simulink library "Solar_Radiation_Sensor"  (R2018b)
settings: Solver=ode45  StartTime=0.0  StopTime=10.0  RelTol=1e-3  EnableMultiTasking=on
settings Model: Creator=lena.frank  LastModifiedBy=P41573
settings DataIOCC: LimitDataPoints=on  SaveFormat=Array  SignalLoggingSaveFormat=ModelDataLogs
settings OptimizationCC: ExpressionDepthLimit=2147483647  LifeSpan=inf
settings DebuggingCC: UnderspecifiedInitializationDetection=Classic  MergeDetectMultiDrivingBlocksExec=none  SolverPrmCheckMsg=warning  FcnCallInpInsideContextMsg=warning  StateNameClashWarn=warning  SFUnexpectedBacktrackingDiag=warning  SFNoUnconditionalDefaultTransitionDiag=warning  SFExecutionAtInitializationDiag=none
settings HardwareCC: ProdBitPerPointer=32  ProdBitPerSizeT=32  ProdBitPerPtrDiffT=32  ProdLargestAtomicFloat=None  ProdIntDivRoundTo=Undefined  ProdEndianess=Unspecified  ProdWordSize=32  ProdHWDeviceType=32-bit Generic
settings ModelReferenceCC: PropagateSignalLabelsOutOfModel=off
settings SFSimCC: SimUseLocalCustomCode=off
settings RTWCC: RTWUseLocalCustomCode=off
settings CodeAppCC: StateflowObjectComments=on
settings GRTTargetCC: TargetLangStandard=C89/C90 (ANSI)  GeneratePreprocessorConditionals=Disable all  CombineOutputUpdateFcns=off  GRTInterface=on
settings ConfigComp: CovMetricSettings=dw  CovHtmlReporting=on  CovSaveCumulativeToWorkspaceVar=on  CovSaveSingleToWorkspaceVar=on  CovExternalEMLEnable=off

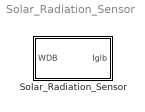
== system Solar_Radiation_Sensor ==
  Solar_Radiation_Sensor : Subsystem  mask(measure solar radiation){rad=diffuse, rad_typ=normal to the beam radiation}
      mask prompts: rad "measured radiation"; rad_typ "orientation of the sensor"
      mask help:
      | Extracts the solar radiation in W/m² from the weather data vector.
      |
      | WARNING:
      | For old weather data vectors, their is only one type of tsolar radiation.
      mask init:
      | if (rad_typ == 1)
      |     if (rad == 1)
      |         vector = [3];
      |     elseif (rad == 2)
      |         vector = [4];
      |     else
      |         vector = [3 4];
      |     end
      | else
      |     if (rad == 1)
      |         vector = [16];
      |     elseif (rad == 2)
      |         vector = [17];
      |     else
      |         vector = [16 17];
      |     end
      | end
      mask Help: web(fullfile(path_carnot('help'),'Solar_Radiation_Sensor.html'),'-helpbrowser')
      mask TypeOptions rad: direct | diffuse | global
      mask TypeOptions rad_typ: normal to the beam radiation | fixed (horizontal or inclined)

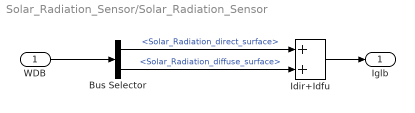
== system Solar_Radiation_Sensor/Solar_Radiation_Sensor ==
  WDB : Inport
  Bus Selector : BusSelector  OutputSignals=Solar_Radiation_direct_surface,Solar_Radiation_diffuse_surface
  Idir+Idfu : Sum  Inputs=2  SaturateOnIntegerOverflow=on  InputSameDT=on  OutDataTypeStr=Inherit: Same as first input
  Iglb : Outport
  wires:
  Bus Selector/2 -> Idir+Idfu/2  "<Solar_Radiation_diffuse_surface>"
  Idir+Idfu/1 -> Iglb/1
  WDB/1 -> Bus Selector/1
  Bus Selector/1 -> Idir+Idfu/1  "<Solar_Radiation_direct_surface>"
